simulink model "main_model"  (R2023a)
settings: Solver=ode15s  StartTime=0.0  StopTime=4  FixedStep=0.0001  RelTol=1e-3  AbsTol=1e-3  EnableMultiTasking=on
model workspace (MAT data in the model file):
  C_Gimbal = 0.5
  C_IAP = 0.01
  K_Gimbal = 0
  K_IAP = 200
  a = 1
  b = 1
  muscle_color = [0 0 1]
  muscle_radius = 1
undefined symbols (not defined in the file): X, Y, Z
libraries: nesl_utility x346, sm_lib x329, simulink_extras x33
(part 8 of 11)

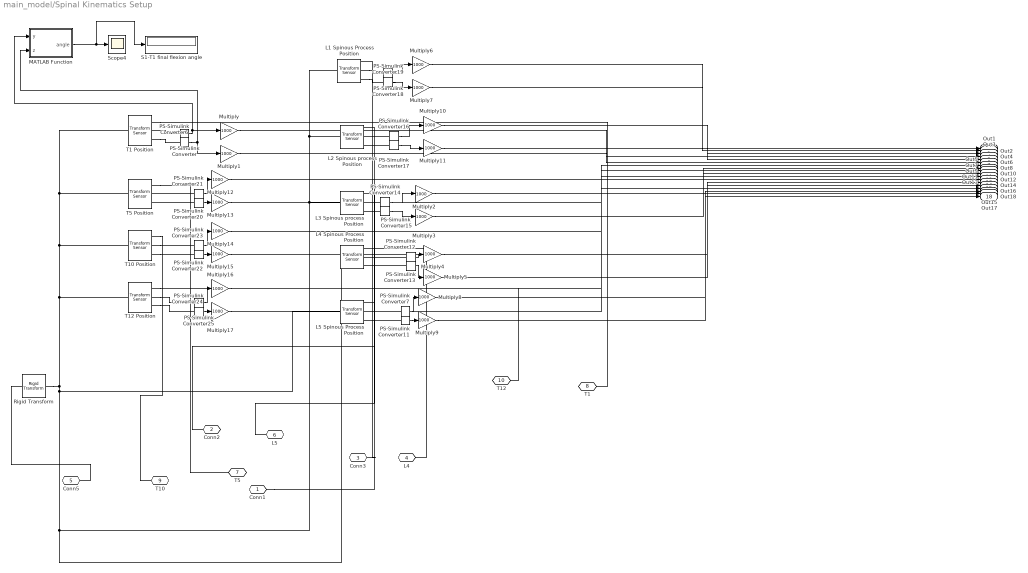
== system main_model/Spinal Kinematics Setup ==
  L1 Spinous Process Position : sm_lib/Frames and Transforms/Transform Sensor  MeasurementFrame=World  RotationSequence=XYX  SenseAngle=off  SenseAxis=off  SenseQ=off  SenseR=off  SenseRotationSequence=off  SenseOmegaX=off  SenseOmegaY=off  SenseOmegaZ=off  SenseQDot=off  SenseRDot=off  SenseRotationSequenceDot=off  SenseAlphaX=off  SenseAlphaY=off  SenseAlphaZ=off  SenseQDDot=off  SenseRDDot=off  SenseX=off  SenseY=on  SenseZ=on  SenseRad=off  SenseAzim=off  SenseDist=off  SenseInc=off  SenseXDot=off  SenseYDot=off  SenseZDot=off  SenseRadDot=off  SenseAzimDot=off  SenseDistDot=off  SenseIncDot=off  SenseXDDot=off  SenseYDDot=off  SenseZDDot=off  SenseRadDDot=off  SenseAzimDDot=off  SenseDistDDot=off  SenseIncDDot=off
  L2 Spinous process Position : sm_lib/Frames and Transforms/Transform Sensor  MeasurementFrame=World  RotationSequence=XYX  SenseAngle=off  SenseAxis=off  SenseQ=off  SenseR=off  SenseRotationSequence=off  SenseOmegaX=off  SenseOmegaY=off  SenseOmegaZ=off  SenseQDot=off  SenseRDot=off  SenseRotationSequenceDot=off  SenseAlphaX=off  SenseAlphaY=off  SenseAlphaZ=off  SenseQDDot=off  SenseRDDot=off  SenseX=off  SenseY=on  SenseZ=on  SenseRad=off  SenseAzim=off  SenseDist=off  SenseInc=off  SenseXDot=off  SenseYDot=off  SenseZDot=off  SenseRadDot=off  SenseAzimDot=off  SenseDistDot=off  SenseIncDot=off  SenseXDDot=off  SenseYDDot=off  SenseZDDot=off  SenseRadDDot=off  SenseAzimDDot=off  SenseDistDDot=off  SenseIncDDot=off
  L3 Spinous process Position : sm_lib/Frames and Transforms/Transform Sensor  MeasurementFrame=World  RotationSequence=XYX  SenseAngle=off  SenseAxis=off  SenseQ=off  SenseR=off  SenseRotationSequence=off  SenseOmegaX=off  SenseOmegaY=off  SenseOmegaZ=off  SenseQDot=off  SenseRDot=off  SenseRotationSequenceDot=off  SenseAlphaX=off  SenseAlphaY=off  SenseAlphaZ=off  SenseQDDot=off  SenseRDDot=off  SenseX=off  SenseY=on  SenseZ=on  SenseRad=off  SenseAzim=off  SenseDist=off  SenseInc=off  SenseXDot=off  SenseYDot=off  SenseZDot=off  SenseRadDot=off  SenseAzimDot=off  SenseDistDot=off  SenseIncDot=off  SenseXDDot=off  SenseYDDot=off  SenseZDDot=off  SenseRadDDot=off  SenseAzimDDot=off  SenseDistDDot=off  SenseIncDDot=off
  L4 Spinous Process Position : sm_lib/Frames and Transforms/Transform Sensor  MeasurementFrame=World  RotationSequence=XYX  SenseAngle=off  SenseAxis=off  SenseQ=off  SenseR=off  SenseRotationSequence=off  SenseOmegaX=off  SenseOmegaY=off  SenseOmegaZ=off  SenseQDot=off  SenseRDot=off  SenseRotationSequenceDot=off  SenseAlphaX=off  SenseAlphaY=off  SenseAlphaZ=off  SenseQDDot=off  SenseRDDot=off  SenseX=off  SenseY=on  SenseZ=on  SenseRad=off  SenseAzim=off  SenseDist=off  SenseInc=off  SenseXDot=off  SenseYDot=off  SenseZDot=off  SenseRadDot=off  SenseAzimDot=off  SenseDistDot=off  SenseIncDot=off  SenseXDDot=off  SenseYDDot=off  SenseZDDot=off  SenseRadDDot=off  SenseAzimDDot=off  SenseDistDDot=off  SenseIncDDot=off
  L5 Spinous Process Position : sm_lib/Frames and Transforms/Transform Sensor  MeasurementFrame=World  RotationSequence=XYX  SenseAngle=off  SenseAxis=off  SenseQ=off  SenseR=off  SenseRotationSequence=off  SenseOmegaX=off  SenseOmegaY=off  SenseOmegaZ=off  SenseQDot=off  SenseRDot=off  SenseRotationSequenceDot=off  SenseAlphaX=off  SenseAlphaY=off  SenseAlphaZ=off  SenseQDDot=off  SenseRDDot=off  SenseX=off  SenseY=on  SenseZ=on  SenseRad=off  SenseAzim=off  SenseDist=off  SenseInc=off  SenseXDot=off  SenseYDot=off  SenseZDot=off  SenseRadDot=off  SenseAzimDot=off  SenseDistDot=off  SenseIncDot=off  SenseXDDot=off  SenseYDDot=off  SenseZDDot=off  SenseRadDDot=off  SenseAzimDDot=off  SenseDistDDot=off  SenseIncDDot=off
  MATLAB Function : MATLAB Function  TreatAsAtomicUnit=on
  Multiply{,1..17} (18 alike) : Gain  Gain=1000
  PS-Simulink Converter{,6..7,11..25} (18 alike) : nesl_utility/PS-Simulink Converter  PhysicalDomain=network_engine_domain  SubClassName=ps_output  LeftPortType=input  RightPortType=output  PseudoPeriodic=off  Frequencies=[]  VectorFormat=inherit  Unit=inherit  AffineConversion=off
  Rigid Transform : sm_lib/Frames and Transforms/Rigid Transform  TranslationMethod=Cartesian  TranslationStandardOffset=0  TranslationStandardOffsetUnits=m  TranslationStandardAxis=+Z  TranslationCartesianOffset=[0 0 0]  TranslationCartesianOffsetUnits=mm  TranslationROffset=0  TranslationROffsetUnits=m  TranslationZOffset=0  TranslationZOffsetUnits=m  TranslationThetaOffset=0  TranslationThetaOffsetUnits=deg  RotationMethod=None  RotationAngleUnits=deg  RotationStandardAxis=+Z  RotationAngle=0.0  RotationArbitraryAxis=[0 0 1]  FollAlignAxisA=+X  BaseAlignAxisA=+Y  FollAlignAxisB=+Y  BaseAlignAxisB=+Z  RotationSequenceAxes=FollowerAxes  RotationSequence=XYX  RotationSequenceAngles=[0 0 0]  RotationSequenceAnglesUnits=deg  RotationMatrix=[1 0 0; 0 1 0; 0 0 1]  Quaternion=[1 0 0 0]
  S1-T1 final flexion angle : Display
  Scope4 : Scope
  T1 Position : sm_lib/Frames and Transforms/Transform Sensor  MeasurementFrame=World  RotationSequence=XYX  SenseAngle=off  SenseAxis=off  SenseQ=off  SenseR=off  SenseRotationSequence=off  SenseOmegaX=off  SenseOmegaY=off  SenseOmegaZ=off  SenseQDot=off  SenseRDot=off  SenseRotationSequenceDot=off  SenseAlphaX=off  SenseAlphaY=off  SenseAlphaZ=off  SenseQDDot=off  SenseRDDot=off  SenseX=off  SenseY=on  SenseZ=on  SenseRad=off  SenseAzim=off  SenseDist=off  SenseInc=off  SenseXDot=off  SenseYDot=off  SenseZDot=off  SenseRadDot=off  SenseAzimDot=off  SenseDistDot=off  SenseIncDot=off  SenseXDDot=off  SenseYDDot=off  SenseZDDot=off  SenseRadDDot=off  SenseAzimDDot=off  SenseDistDDot=off  SenseIncDDot=off
  T10 Position : sm_lib/Frames and Transforms/Transform Sensor  MeasurementFrame=World  RotationSequence=XYX  SenseAngle=off  SenseAxis=off  SenseQ=off  SenseR=off  SenseRotationSequence=off  SenseOmegaX=off  SenseOmegaY=off  SenseOmegaZ=off  SenseQDot=off  SenseRDot=off  SenseRotationSequenceDot=off  SenseAlphaX=off  SenseAlphaY=off  SenseAlphaZ=off  SenseQDDot=off  SenseRDDot=off  SenseX=off  SenseY=on  SenseZ=on  SenseRad=off  SenseAzim=off  SenseDist=off  SenseInc=off  SenseXDot=off  SenseYDot=off  SenseZDot=off  SenseRadDot=off  SenseAzimDot=off  SenseDistDot=off  SenseIncDot=off  SenseXDDot=off  SenseYDDot=off  SenseZDDot=off  SenseRadDDot=off  SenseAzimDDot=off  SenseDistDDot=off  SenseIncDDot=off
  T12 Position : sm_lib/Frames and Transforms/Transform Sensor  MeasurementFrame=World  RotationSequence=XYX  SenseAngle=off  SenseAxis=off  SenseQ=off  SenseR=off  SenseRotationSequence=off  SenseOmegaX=off  SenseOmegaY=off  SenseOmegaZ=off  SenseQDot=off  SenseRDot=off  SenseRotationSequenceDot=off  SenseAlphaX=off  SenseAlphaY=off  SenseAlphaZ=off  SenseQDDot=off  SenseRDDot=off  SenseX=off  SenseY=on  SenseZ=on  SenseRad=off  SenseAzim=off  SenseDist=off  SenseInc=off  SenseXDot=off  SenseYDot=off  SenseZDot=off  SenseRadDot=off  SenseAzimDot=off  SenseDistDot=off  SenseIncDot=off  SenseXDDot=off  SenseYDDot=off  SenseZDDot=off  SenseRadDDot=off  SenseAzimDDot=off  SenseDistDDot=off  SenseIncDDot=off
  T5 Position : sm_lib/Frames and Transforms/Transform Sensor  MeasurementFrame=World  RotationSequence=XYX  SenseAngle=off  SenseAxis=off  SenseQ=off  SenseR=off  SenseRotationSequence=off  SenseOmegaX=off  SenseOmegaY=off  SenseOmegaZ=off  SenseQDot=off  SenseRDot=off  SenseRotationSequenceDot=off  SenseAlphaX=off  SenseAlphaY=off  SenseAlphaZ=off  SenseQDDot=off  SenseRDDot=off  SenseX=off  SenseY=on  SenseZ=on  SenseRad=off  SenseAzim=off  SenseDist=off  SenseInc=off  SenseXDot=off  SenseYDot=off  SenseZDot=off  SenseRadDot=off  SenseAzimDot=off  SenseDistDot=off  SenseIncDot=off  SenseXDDot=off  SenseYDDot=off  SenseZDDot=off  SenseRadDDot=off  SenseAzimDDot=off  SenseDistDDot=off  SenseIncDDot=off
  Conn1 : PMIOPort  Side=Right
  Conn2 : PMIOPort  Port=2  Side=Right
  Conn3 : PMIOPort  Port=3  Side=Right
  L4 : PMIOPort  Port=4  Side=Right
  Conn5 : PMIOPort  Port=5  Side=Left
  L5 : PMIOPort  Port=6  Side=Right
  T5 : PMIOPort  Port=7  Side=Right
  T1 : PMIOPort  Port=8  Side=Right
  T10 : PMIOPort  Port=9  Side=Right
  T12 : PMIOPort  Port=10  Side=Right
  Out1 : Outport
  Out2 : Outport  Port=2
  Out3 : Outport  Port=3
  Out4 : Outport  Port=4
  Out5 : Outport  Port=5
  Out6 : Outport  Port=6
  Out7 : Outport  Port=7
  Out8 : Outport  Port=8
  Out9 : Outport  Port=9
  Out10 : Outport  Port=10
  Out11 : Outport  Port=11
  Out12 : Outport  Port=12
  Out13 : Outport  Port=13
  Out14 : Outport  Port=14
  Out15 : Outport  Port=15
  Out16 : Outport  Port=16
  Out17 : Outport  Port=17
  Out18 : Outport  Port=18
  wires:
  Multiply9/1 -> Out18/1
  Multiply17/1 -> Out17/1
  Multiply5/1 -> Out14/1
  Multiply12/1 -> Out7/1
  Multiply2/1 -> Out8/1
  Multiply10/1 -> Out3/1
  Multiply13/1 -> Out9/1
  Multiply6/1 -> Out1/1
  Multiply4/1 -> Out13/1
  PS-Simulink Converter7/1 -> Multiply8/1
  PS-Simulink Converter13/1 -> Multiply5/1
  Multiply11/1 -> Out5/1
  Multiply8/1 -> Out16/1
  Multiply/1 -> Out4/1
  Multiply16/1 -> Out15/1
  PS-Simulink Converter24/1 -> Multiply17/1
  Multiply15/1 -> Out12/1
  Multiply7/1 -> Out2/1
  PS-Simulink Converter22/1 -> Multiply15/1
  PS-Simulink Converter23/1 -> Multiply14/1
  PS-Simulink Converter15/1 -> Multiply3/1
  PS-Simulink Converter20/1 -> Multiply13/1
  PS-Simulink Converter11/1 -> Multiply9/1
  PS-Simulink Converter14/1 -> Multiply2/1
  Multiply14/1 -> Out11/1
  PS-Simulink Converter21/1 -> Multiply12/1
  PS-Simulink Converter18/1 -> Multiply6/1
  Multiply1/1 -> Out6/1
  PS-Simulink Converter16/1 -> Multiply10/1
  PS-Simulink Converter17/1 -> Multiply11/1
  Multiply3/1 -> Out10/1
  PS-Simulink Converter25/1 -> Multiply16/1
  PS-Simulink Converter12/1 -> Multiply4/1
  PS-Simulink Converter19/1 -> Multiply7/1
  MATLAB Function/1(angle) -> Scope4/1, S1-T1 final flexion angle/1
  PS-Simulink Converter/1 -> MATLAB Function/1(y), Multiply/1
  PS-Simulink Converter6/1 -> Multiply1/1, MATLAB Function/2(z)
  connections:
  L4 Spinous Process Position/RConn1 -- L4/RConn1
  T10 Position/RConn1 -- T10/RConn1
  L1 Spinous Process Position/RConn2 -- PS-Simulink Converter18/LConn1
  T5 Position/RConn1 -- T5/RConn1
  PS-Simulink Converter21/LConn1 -- T5 Position/RConn2
  L3 Spinous process Position/RConn2 -- PS-Simulink Converter14/LConn1
  T10 Position/RConn3 -- PS-Simulink Converter22/LConn1
  T1 Position/RConn3 -- PS-Simulink Converter6/LConn1
  PS-Simulink Converter20/LConn1 -- T5 Position/RConn3
  Conn1/RConn1 -- L2 Spinous process Position/RConn1
  L1 Spinous Process Position/RConn3 -- PS-Simulink Converter19/LConn1
  Rigid Transform/LConn1 -- Conn5/RConn1
  L2 Spinous process Position/RConn3 -- PS-Simulink Converter17/LConn1
  T1 Position/RConn2 -- PS-Simulink Converter/LConn1
  L5 Spinous Process Position/RConn1 -- L5/RConn1
  T10 Position/RConn2 -- PS-Simulink Converter23/LConn1
  L5 Spinous Process Position/RConn2 -- PS-Simulink Converter7/LConn1
  L3 Spinous process Position/RConn1 -- Conn2/RConn1
  T12 Position/RConn3 -- PS-Simulink Converter24/LConn1
  T12 Position/RConn2 -- PS-Simulink Converter25/LConn1
  Conn3/RConn1 -- L1 Spinous Process Position/RConn1
  L4 Spinous Process Position/LConn1 -- L3 Spinous process Position/LConn1 -- L2 Spinous process Position/LConn1 -- L1 Spinous Process Position/LConn1 -- L5 Spinous Process Position/LConn1 -- Rigid Transform/RConn1 -- T12 Position/LConn1 -- T10 Position/LConn1 -- T5 Position/LConn1 -- T1 Position/LConn1
  L5 Spinous Process Position/RConn3 -- PS-Simulink Converter11/LConn1
  L3 Spinous process Position/RConn3 -- PS-Simulink Converter15/LConn1
  T1 Position/RConn1 -- T1/RConn1
  L4 Spinous Process Position/RConn2 -- PS-Simulink Converter12/LConn1
  T12 Position/RConn1 -- T12/RConn1
  L4 Spinous Process Position/RConn3 -- PS-Simulink Converter13/LConn1
  L2 Spinous process Position/RConn2 -- PS-Simulink Converter16/LConn1

== system main_model/L1/AR torque feedback L4 ==
  Constant : Constant  Value=0.7
  Constant1 : Constant  Value=0.7
  Gain5 : Gain  Gain=-1
  PS-Simulink Converter9 : nesl_utility/PS-Simulink Converter  PhysicalDomain=network_engine_domain  SubClassName=ps_output  LeftPortType=input  RightPortType=output  PseudoPeriodic=off  Frequencies=[]  VectorFormat=1-D array  Unit=inherit  AffineConversion=off
  Radians to Degrees : simulink_extras/Transformations/Radians to Degrees
  Simulink-PS Converter6 : nesl_utility/Simulink-PS Converter  PhysicalDomain=network_engine_domain  SubClassName=ps_input  LeftPortType=input  RightPortType=output  PseudoPeriodic=off  Frequencies=[]  NoiseDistribution=none  NoiseParameters=[]  Unit=1  AffineConversion=off  FilteringAndDerivatives=provide  SimscapeFilterOrder=1  InputFilterTimeConstant=0.001  UdotUserProvided=0
  peacewise torque profile5 : MATLAB Function  TreatAsAtomicUnit=on
  AR rot : PMIOPort  Side=Left
  AR torque : PMIOPort  Port=2  Side=Right
  wires:
  Constant1/1 -> peacewise torque profile5/3(b)
  Constant/1 -> peacewise torque profile5/2(a)
  Radians to Degrees/1 -> peacewise torque profile5/1(u)
  Gain5/1 -> Simulink-PS Converter6/1
  peacewise torque profile5/1(torque) -> Gain5/1
  PS-Simulink Converter9/1 -> Radians to Degrees/1
  connections:
  AR torque/RConn1 -- Simulink-PS Converter6/RConn1
  PS-Simulink Converter9/LConn1 -- AR rot/RConn1

== system main_model/L1/FE torque feedback L4 ==
  Constant : Constant  Value=a
  Constant1 : Constant  Value=b
  Gain1 : Gain  Gain=-1
  Gain7 : Gain
  PS-Simulink Converter5 : nesl_utility/PS-Simulink Converter  PhysicalDomain=network_engine_domain  SubClassName=ps_output  LeftPortType=input  RightPortType=output  PseudoPeriodic=off  Frequencies=[]  VectorFormat=1-D array  Unit=inherit  AffineConversion=off
  Radians to Degrees : simulink_extras/Transformations/Radians to Degrees
  Simulink-PS Converter4 : nesl_utility/Simulink-PS Converter  PhysicalDomain=network_engine_domain  SubClassName=ps_input  LeftPortType=input  RightPortType=output  PseudoPeriodic=off  Frequencies=[]  NoiseDistribution=none  NoiseParameters=[]  Unit=1  AffineConversion=off  FilteringAndDerivatives=provide  SimscapeFilterOrder=1  InputFilterTimeConstant=0.001  UdotUserProvided=0
  peacewise torque profile1 : MATLAB Function  TreatAsAtomicUnit=on
  FE rot : PMIOPort  Side=Left
  FE torque : PMIOPort  Port=2  Side=Right
  wires:
  Constant1/1 -> peacewise torque profile1/3(b)
  Constant/1 -> peacewise torque profile1/2(a)
  Gain1/1 -> peacewise torque profile1/1(u)
  Radians to Degrees/1 -> Gain1/1
  Gain7/1 -> Simulink-PS Converter4/1
  peacewise torque profile1/1(torque) -> Gain7/1
  PS-Simulink Converter5/1 -> Radians to Degrees/1
  connections:
  FE torque/RConn1 -- Simulink-PS Converter4/RConn1
  FE rot/RConn1 -- PS-Simulink Converter5/LConn1

== system main_model/L1/LB torque feedback L4 ==
  Constant : Constant  Value=a
  Constant1 : Constant  Value=b
  Gain4 : Gain  Gain=-1
  PS-Simulink Converter8 : nesl_utility/PS-Simulink Converter  PhysicalDomain=network_engine_domain  SubClassName=ps_output  LeftPortType=input  RightPortType=output  PseudoPeriodic=off  Frequencies=[]  VectorFormat=1-D array  Unit=inherit  AffineConversion=off
  Radians to Degrees : simulink_extras/Transformations/Radians to Degrees
  Simulink-PS Converter5 : nesl_utility/Simulink-PS Converter  PhysicalDomain=network_engine_domain  SubClassName=ps_input  LeftPortType=input  RightPortType=output  PseudoPeriodic=off  Frequencies=[]  NoiseDistribution=none  NoiseParameters=[]  Unit=1  AffineConversion=off  FilteringAndDerivatives=provide  SimscapeFilterOrder=1  InputFilterTimeConstant=0.001  UdotUserProvided=0
  peacewise torque profile4 : MATLAB Function  TreatAsAtomicUnit=on
  LB rot : PMIOPort  Side=Left
  LB torque : PMIOPort  Port=2  Side=Right
  wires:
  Radians to Degrees/1 -> peacewise torque profile4/1(u)
  Constant1/1 -> peacewise torque profile4/3(b)
  Constant/1 -> peacewise torque profile4/2(a)
  peacewise torque profile4/1(torque) -> Gain4/1
  PS-Simulink Converter8/1 -> Radians to Degrees/1
  Gain4/1 -> Simulink-PS Converter5/1
  connections:
  LB rot/RConn1 -- PS-Simulink Converter8/LConn1
  Simulink-PS Converter5/RConn1 -- LB torque/RConn1

== system main_model/L2/AR torque feedback L4 ==
  Constant : Constant  Value=0.7
  Constant1 : Constant  Value=0.7
  Gain5 : Gain  Gain=-1
  PS-Simulink Converter9 : nesl_utility/PS-Simulink Converter  PhysicalDomain=network_engine_domain  SubClassName=ps_output  LeftPortType=input  RightPortType=output  PseudoPeriodic=off  Frequencies=[]  VectorFormat=1-D array  Unit=inherit  AffineConversion=off
  Radians to Degrees : simulink_extras/Transformations/Radians to Degrees
  Simulink-PS Converter6 : nesl_utility/Simulink-PS Converter  PhysicalDomain=network_engine_domain  SubClassName=ps_input  LeftPortType=input  RightPortType=output  PseudoPeriodic=off  Frequencies=[]  NoiseDistribution=none  NoiseParameters=[]  Unit=1  AffineConversion=off  FilteringAndDerivatives=provide  SimscapeFilterOrder=1  InputFilterTimeConstant=0.001  UdotUserProvided=0
  peacewise torque profile5 : MATLAB Function  TreatAsAtomicUnit=on
  AR rot : PMIOPort  Side=Left
  AR torque : PMIOPort  Port=2  Side=Right
  wires:
  Constant1/1 -> peacewise torque profile5/3(b)
  Constant/1 -> peacewise torque profile5/2(a)
  Radians to Degrees/1 -> peacewise torque profile5/1(u)
  PS-Simulink Converter9/1 -> Radians to Degrees/1
  peacewise torque profile5/1(torque) -> Gain5/1
  Gain5/1 -> Simulink-PS Converter6/1
  connections:
  PS-Simulink Converter9/LConn1 -- AR rot/RConn1
  AR torque/RConn1 -- Simulink-PS Converter6/RConn1

== system main_model/L2/FE torque feedback L4 ==
  Constant : Constant  Value=a
  Constant1 : Constant  Value=b
  Gain1 : Gain  Gain=-1
  Gain7 : Gain
  PS-Simulink Converter5 : nesl_utility/PS-Simulink Converter  PhysicalDomain=network_engine_domain  SubClassName=ps_output  LeftPortType=input  RightPortType=output  PseudoPeriodic=off  Frequencies=[]  VectorFormat=1-D array  Unit=inherit  AffineConversion=off
  Radians to Degrees : simulink_extras/Transformations/Radians to Degrees
  Simulink-PS Converter4 : nesl_utility/Simulink-PS Converter  PhysicalDomain=network_engine_domain  SubClassName=ps_input  LeftPortType=input  RightPortType=output  PseudoPeriodic=off  Frequencies=[]  NoiseDistribution=none  NoiseParameters=[]  Unit=1  AffineConversion=off  FilteringAndDerivatives=provide  SimscapeFilterOrder=1  InputFilterTimeConstant=0.001  UdotUserProvided=0
  peacewise torque profile1 : MATLAB Function  TreatAsAtomicUnit=on
  FE rot : PMIOPort  Side=Left
  FE torque : PMIOPort  Port=2  Side=Right
  wires:
  Gain1/1 -> peacewise torque profile1/1(u)
  Constant1/1 -> peacewise torque profile1/3(b)
  Constant/1 -> peacewise torque profile1/2(a)
  PS-Simulink Converter5/1 -> Radians to Degrees/1
  Radians to Degrees/1 -> Gain1/1
  peacewise torque profile1/1(torque) -> Gain7/1
  Gain7/1 -> Simulink-PS Converter4/1
  connections:
  FE rot/RConn1 -- PS-Simulink Converter5/LConn1
  FE torque/RConn1 -- Simulink-PS Converter4/RConn1

== system main_model/L2/LB torque feedback L4 ==
  Constant : Constant  Value=a
  Constant1 : Constant  Value=b
  Gain4 : Gain  Gain=-1
  PS-Simulink Converter8 : nesl_utility/PS-Simulink Converter  PhysicalDomain=network_engine_domain  SubClassName=ps_output  LeftPortType=input  RightPortType=output  PseudoPeriodic=off  Frequencies=[]  VectorFormat=1-D array  Unit=inherit  AffineConversion=off
  Radians to Degrees : simulink_extras/Transformations/Radians to Degrees
  Simulink-PS Converter5 : nesl_utility/Simulink-PS Converter  PhysicalDomain=network_engine_domain  SubClassName=ps_input  LeftPortType=input  RightPortType=output  PseudoPeriodic=off  Frequencies=[]  NoiseDistribution=none  NoiseParameters=[]  Unit=1  AffineConversion=off  FilteringAndDerivatives=provide  SimscapeFilterOrder=1  InputFilterTimeConstant=0.001  UdotUserProvided=0
  peacewise torque profile4 : MATLAB Function  TreatAsAtomicUnit=on
  LB rot : PMIOPort  Side=Left
  LB torque : PMIOPort  Port=2  Side=Right
  wires:
  Radians to Degrees/1 -> peacewise torque profile4/1(u)
  Constant1/1 -> peacewise torque profile4/3(b)
  Constant/1 -> peacewise torque profile4/2(a)
  Gain4/1 -> Simulink-PS Converter5/1
  PS-Simulink Converter8/1 -> Radians to Degrees/1
  peacewise torque profile4/1(torque) -> Gain4/1
  connections:
  Simulink-PS Converter5/RConn1 -- LB torque/RConn1
  LB rot/RConn1 -- PS-Simulink Converter8/LConn1

== system main_model/L3/AR torque feedback L4 ==
  Constant : Constant  Value=0.7
  Constant1 : Constant  Value=0.7
  Gain5 : Gain  Gain=-1
  PS-Simulink Converter9 : nesl_utility/PS-Simulink Converter  PhysicalDomain=network_engine_domain  SubClassName=ps_output  LeftPortType=input  RightPortType=output  PseudoPeriodic=off  Frequencies=[]  VectorFormat=1-D array  Unit=inherit  AffineConversion=off
  Radians to Degrees : simulink_extras/Transformations/Radians to Degrees
  Simulink-PS Converter6 : nesl_utility/Simulink-PS Converter  PhysicalDomain=network_engine_domain  SubClassName=ps_input  LeftPortType=input  RightPortType=output  PseudoPeriodic=off  Frequencies=[]  NoiseDistribution=none  NoiseParameters=[]  Unit=1  AffineConversion=off  FilteringAndDerivatives=provide  SimscapeFilterOrder=1  InputFilterTimeConstant=0.001  UdotUserProvided=0
  peacewise torque profile5 : MATLAB Function  TreatAsAtomicUnit=on
  AR rot : PMIOPort  Side=Left
  AR torque : PMIOPort  Port=2  Side=Right
  wires:
  Constant1/1 -> peacewise torque profile5/3(b)
  Constant/1 -> peacewise torque profile5/2(a)
  Radians to Degrees/1 -> peacewise torque profile5/1(u)
  PS-Simulink Converter9/1 -> Radians to Degrees/1
  Gain5/1 -> Simulink-PS Converter6/1
  peacewise torque profile5/1(torque) -> Gain5/1
  connections:
  AR torque/RConn1 -- Simulink-PS Converter6/RConn1
  PS-Simulink Converter9/LConn1 -- AR rot/RConn1

== system main_model/L3/FE torque feedback L4 ==
  Constant : Constant  Value=a
  Constant1 : Constant  Value=b
  Gain1 : Gain  Gain=-1
  Gain7 : Gain
  PS-Simulink Converter5 : nesl_utility/PS-Simulink Converter  PhysicalDomain=network_engine_domain  SubClassName=ps_output  LeftPortType=input  RightPortType=output  PseudoPeriodic=off  Frequencies=[]  VectorFormat=1-D array  Unit=inherit  AffineConversion=off
  Radians to Degrees : simulink_extras/Transformations/Radians to Degrees
  Simulink-PS Converter4 : nesl_utility/Simulink-PS Converter  PhysicalDomain=network_engine_domain  SubClassName=ps_input  LeftPortType=input  RightPortType=output  PseudoPeriodic=off  Frequencies=[]  NoiseDistribution=none  NoiseParameters=[]  Unit=1  AffineConversion=off  FilteringAndDerivatives=provide  SimscapeFilterOrder=1  InputFilterTimeConstant=0.001  UdotUserProvided=0
  peacewise torque profile1 : MATLAB Function  TreatAsAtomicUnit=on
  FE rot : PMIOPort  Side=Left
  FE torque : PMIOPort  Port=2  Side=Right
  wires:
  Gain1/1 -> peacewise torque profile1/1(u)
  Constant1/1 -> peacewise torque profile1/3(b)
  Constant/1 -> peacewise torque profile1/2(a)
  PS-Simulink Converter5/1 -> Radians to Degrees/1
  Radians to Degrees/1 -> Gain1/1
  Gain7/1 -> Simulink-PS Converter4/1
  peacewise torque profile1/1(torque) -> Gain7/1
  connections:
  FE torque/RConn1 -- Simulink-PS Converter4/RConn1
  FE rot/RConn1 -- PS-Simulink Converter5/LConn1

== system main_model/L3/LB torque feedback L4 ==
  Constant : Constant  Value=a
  Constant1 : Constant  Value=b
  Gain4 : Gain  Gain=-1
  PS-Simulink Converter8 : nesl_utility/PS-Simulink Converter  PhysicalDomain=network_engine_domain  SubClassName=ps_output  LeftPortType=input  RightPortType=output  PseudoPeriodic=off  Frequencies=[]  VectorFormat=1-D array  Unit=inherit  AffineConversion=off
  Radians to Degrees : simulink_extras/Transformations/Radians to Degrees
  Simulink-PS Converter5 : nesl_utility/Simulink-PS Converter  PhysicalDomain=network_engine_domain  SubClassName=ps_input  LeftPortType=input  RightPortType=output  PseudoPeriodic=off  Frequencies=[]  NoiseDistribution=none  NoiseParameters=[]  Unit=1  AffineConversion=off  FilteringAndDerivatives=provide  SimscapeFilterOrder=1  InputFilterTimeConstant=0.001  UdotUserProvided=0
  peacewise torque profile4 : MATLAB Function  TreatAsAtomicUnit=on
  LB rot : PMIOPort  Side=Left
  LB torque : PMIOPort  Port=2  Side=Right
  wires:
  Radians to Degrees/1 -> peacewise torque profile4/1(u)
  Constant1/1 -> peacewise torque profile4/3(b)
  Constant/1 -> peacewise torque profile4/2(a)
  peacewise torque profile4/1(torque) -> Gain4/1
  PS-Simulink Converter8/1 -> Radians to Degrees/1
  Gain4/1 -> Simulink-PS Converter5/1
  connections:
  LB rot/RConn1 -- PS-Simulink Converter8/LConn1
  Simulink-PS Converter5/RConn1 -- LB torque/RConn1

== system main_model/L4/AR torque feedback L4 ==
  Constant : Constant  Value=0.7
  Constant1 : Constant  Value=0.7
  Gain5 : Gain  Gain=-1
  PS-Simulink Converter9 : nesl_utility/PS-Simulink Converter  PhysicalDomain=network_engine_domain  SubClassName=ps_output  LeftPortType=input  RightPortType=output  PseudoPeriodic=off  Frequencies=[]  VectorFormat=1-D array  Unit=inherit  AffineConversion=off
  Radians to Degrees : simulink_extras/Transformations/Radians to Degrees
  Simulink-PS Converter6 : nesl_utility/Simulink-PS Converter  PhysicalDomain=network_engine_domain  SubClassName=ps_input  LeftPortType=input  RightPortType=output  PseudoPeriodic=off  Frequencies=[]  NoiseDistribution=none  NoiseParameters=[]  Unit=1  AffineConversion=off  FilteringAndDerivatives=provide  SimscapeFilterOrder=1  InputFilterTimeConstant=0.001  UdotUserProvided=0
  peacewise torque profile5 : MATLAB Function  TreatAsAtomicUnit=on
  AR rot : PMIOPort  Side=Left
  AR torque : PMIOPort  Port=2  Side=Right
  wires:
  Constant1/1 -> peacewise torque profile5/3(b)
  Constant/1 -> peacewise torque profile5/2(a)
  Radians to Degrees/1 -> peacewise torque profile5/1(u)
  PS-Simulink Converter9/1 -> Radians to Degrees/1
  peacewise torque profile5/1(torque) -> Gain5/1
  Gain5/1 -> Simulink-PS Converter6/1
  connections:
  PS-Simulink Converter9/LConn1 -- AR rot/RConn1
  AR torque/RConn1 -- Simulink-PS Converter6/RConn1

== system main_model/L4/FE torque feedback L4 ==
  Constant : Constant  Value=a
  Constant1 : Constant  Value=b
  Gain1 : Gain  Gain=-1
  Gain7 : Gain
  PS-Simulink Converter5 : nesl_utility/PS-Simulink Converter  PhysicalDomain=network_engine_domain  SubClassName=ps_output  LeftPortType=input  RightPortType=output  PseudoPeriodic=off  Frequencies=[]  VectorFormat=1-D array  Unit=inherit  AffineConversion=off
  Radians to Degrees : simulink_extras/Transformations/Radians to Degrees
  Scope : Scope  NumInputPorts=2
  Simulink-PS Converter4 : nesl_utility/Simulink-PS Converter  PhysicalDomain=network_engine_domain  SubClassName=ps_input  LeftPortType=input  RightPortType=output  PseudoPeriodic=off  Frequencies=[]  NoiseDistribution=none  NoiseParameters=[]  Unit=1  AffineConversion=off  FilteringAndDerivatives=provide  SimscapeFilterOrder=1  InputFilterTimeConstant=0.001  UdotUserProvided=0
  peacewise torque profile1 : MATLAB Function  TreatAsAtomicUnit=on
  FE rot : PMIOPort  Side=Left
  FE torque : PMIOPort  Port=2  Side=Right
  wires:
  Gain1/1 -> peacewise torque profile1/1(u), Scope/1
  Constant1/1 -> peacewise torque profile1/3(b)
  Constant/1 -> peacewise torque profile1/2(a)
  PS-Simulink Converter5/1 -> Radians to Degrees/1
  Radians to Degrees/1 -> Gain1/1
  peacewise torque profile1/1(torque) -> Gain7/1
  Gain7/1 -> Simulink-PS Converter4/1, Scope/2
  connections:
  FE rot/RConn1 -- PS-Simulink Converter5/LConn1
  FE torque/RConn1 -- Simulink-PS Converter4/RConn1

== system main_model/L4/LB torque feedback L4 ==
  Constant : Constant  Value=a
  Constant1 : Constant  Value=b
  Gain4 : Gain  Gain=-1
  PS-Simulink Converter8 : nesl_utility/PS-Simulink Converter  PhysicalDomain=network_engine_domain  SubClassName=ps_output  LeftPortType=input  RightPortType=output  PseudoPeriodic=off  Frequencies=[]  VectorFormat=1-D array  Unit=inherit  AffineConversion=off
  Radians to Degrees : simulink_extras/Transformations/Radians to Degrees
  Simulink-PS Converter5 : nesl_utility/Simulink-PS Converter  PhysicalDomain=network_engine_domain  SubClassName=ps_input  LeftPortType=input  RightPortType=output  PseudoPeriodic=off  Frequencies=[]  NoiseDistribution=none  NoiseParameters=[]  Unit=1  AffineConversion=off  FilteringAndDerivatives=provide  SimscapeFilterOrder=1  InputFilterTimeConstant=0.001  UdotUserProvided=0
  peacewise torque profile4 : MATLAB Function  TreatAsAtomicUnit=on
  LB rot : PMIOPort  Side=Left
  LB torque : PMIOPort  Port=2  Side=Right
  wires:
  Radians to Degrees/1 -> peacewise torque profile4/1(u)
  Constant1/1 -> peacewise torque profile4/3(b)
  Constant/1 -> peacewise torque profile4/2(a)
  Gain4/1 -> Simulink-PS Converter5/1
  PS-Simulink Converter8/1 -> Radians to Degrees/1
  peacewise torque profile4/1(torque) -> Gain4/1
  connections:
  Simulink-PS Converter5/RConn1 -- LB torque/RConn1
  LB rot/RConn1 -- PS-Simulink Converter8/LConn1

== system main_model/L5/AR torque feedback L5 ==
  Constant : Constant  Value=0.7
  Constant1 : Constant  Value=0.7
  Gain2 : Gain  Gain=-1
  PS-Simulink Converter3 : nesl_utility/PS-Simulink Converter  PhysicalDomain=network_engine_domain  SubClassName=ps_output  LeftPortType=input  RightPortType=output  PseudoPeriodic=off  Frequencies=[]  VectorFormat=1-D array  Unit=inherit  AffineConversion=off
  Radians to Degrees : simulink_extras/Transformations/Radians to Degrees
  Simulink-PS Converter2 : nesl_utility/Simulink-PS Converter  PhysicalDomain=network_engine_domain  SubClassName=ps_input  LeftPortType=input  RightPortType=output  PseudoPeriodic=off  Frequencies=[]  NoiseDistribution=none  NoiseParameters=[]  Unit=1  AffineConversion=off  FilteringAndDerivatives=provide  SimscapeFilterOrder=1  InputFilterTimeConstant=0.001  UdotUserProvided=0
  peacewise torque profile3 : MATLAB Function  TreatAsAtomicUnit=on
  AR rot : PMIOPort  Side=Left
  AR torque : PMIOPort  Port=2  Side=Right
  wires:
  Constant1/1 -> peacewise torque profile3/3(b)
  Constant/1 -> peacewise torque profile3/2(a)
  Radians to Degrees/1 -> peacewise torque profile3/1(u)
  PS-Simulink Converter3/1 -> Radians to Degrees/1
  Gain2/1 -> Simulink-PS Converter2/1
  peacewise torque profile3/1(torque) -> Gain2/1
  connections:
  PS-Simulink Converter3/LConn1 -- AR rot/RConn1
  AR torque/RConn1 -- Simulink-PS Converter2/RConn1

== system main_model/L5/FE torque feedback L5 ==
  Constant : Constant  Value=a
  Constant1 : Constant  Value=b
  Gain1 : Gain  Gain=-1
  Gain6 : Gain
  PS-Simulink Converter : nesl_utility/PS-Simulink Converter  PhysicalDomain=network_engine_domain  SubClassName=ps_output  LeftPortType=input  RightPortType=output  PseudoPeriodic=off  Frequencies=[]  VectorFormat=inherit  Unit=inherit  AffineConversion=off
  Radians to Degrees : simulink_extras/Transformations/Radians to Degrees
  Scope : Scope  NumInputPorts=2
  Simulink-PS Converter3 : nesl_utility/Simulink-PS Converter  PhysicalDomain=network_engine_domain  SubClassName=ps_input  LeftPortType=input  RightPortType=output  PseudoPeriodic=off  Frequencies=[]  NoiseDistribution=none  NoiseParameters=[]  Unit=1  AffineConversion=off  FilteringAndDerivatives=provide  SimscapeFilterOrder=1  InputFilterTimeConstant=0.001  UdotUserProvided=0
  XY Graph : Record  FileSettingsInternal="{\"entries\":[{\"content\":{\"excelSettings\":{\"content\":{},\"type\":\"Streamout.ExcelSettings\"}},\"type\":\"Streamout.FileSettingStorage\",\"uuid\":\"21849821-9f95-4fe4-8d79-13356bbc0b36\"}],\"packageUris\":[\"http://schema.mathworks.com/mf0/streamout_blocks/R2020a\"],\"version\":\"1.0\"}"  Layout=[1 1]  SignalsInternal="{\"entries\":[{\"content\":{\"signals\":[{\"content\":{\"blockPath\":[\"main_model/L5/FE torque feedback L5/XY Graph\"],\"dimensions\":[1],\"domain\":\"main_model/L5/FE torque feedback L5/XY Graph\",\"lineColor\":\"#4dbeee\",\"port\":1,\"signalID\":1772,\"signalName\":\"moment\"},\"type\":\"RecordBlkView.Signal\",\"uuid\":\"63c73282-42d9-4aea-a135-8bf1856202d8\"},{\"content\":{\"blockPath\":[\"main_model/L5/FE torque feedback L5/XY Graph\"],\"dimensions\":[1,1],\"domain\":\"main_model/L5/FE torque feedback L5/XY Graph\",\"lineColor\":\"#a2142f\",\"port\":2,\"signalID\":1775,\"signalName\":\"rot\"},\"type\":\"RecordBlkView.Signal\",\"uuid\":\"2cce2bc2-92f3-4c7e-868c-ac92c3e97ccb\"}]},\"type\":\"RecordBlkView.InputSignals\",\"uuid\":\"b0d75595-b0eb-49bf-926c-fd4db05ca047\"}],\"packageUris\":[\"http://schema.mathworks.com/mf0/streamout_blocks/R2020a\"],\"version\":\"1.0\"}"  VisualizationBindings="{\"xyplotplugin\":{\"info\":[{\"series\":[],\"subplotID\":1}]}}"  CompatibilityTag=XY
  peacewise torque profile (+- 15 deg) : MATLAB Function  TreatAsAtomicUnit=on
  FE torque : PMIOPort  Side=Right
  FE rot : PMIOPort  Port=2  Side=Left
  wires:
  Gain1/1 -> peacewise torque profile (+- 15 deg)/1(u), Scope/2, XY Graph/2  "rot"
  Constant1/1 -> peacewise torque profile (+- 15 deg)/3(b)
  Constant/1 -> peacewise torque profile (+- 15 deg)/2(a)
  PS-Simulink Converter/1 -> Radians to Degrees/1
  Radians to Degrees/1 -> Gain1/1
  peacewise torque profile (+- 15 deg)/1(torque) -> Gain6/1
  Gain6/1 -> Simulink-PS Converter3/1, Scope/1, XY Graph/1  "moment"
  connections:
  Simulink-PS Converter3/RConn1 -- FE torque/RConn1
  FE rot/RConn1 -- PS-Simulink Converter/LConn1

== system main_model/L5/LB torque feedback L5 ==
  Constant : Constant  Value=a
  Constant1 : Constant  Value=b
  Gain1 : Gain  Gain=-1
  PS-Simulink Converter2 : nesl_utility/PS-Simulink Converter  PhysicalDomain=network_engine_domain  SubClassName=ps_output  LeftPortType=input  RightPortType=output  PseudoPeriodic=off  Frequencies=[]  VectorFormat=1-D array  Unit=inherit  AffineConversion=off
  Radians to Degrees : simulink_extras/Transformations/Radians to Degrees
  Simulink-PS Converter1 : nesl_utility/Simulink-PS Converter  PhysicalDomain=network_engine_domain  SubClassName=ps_input  LeftPortType=input  RightPortType=output  PseudoPeriodic=off  Frequencies=[]  NoiseDistribution=none  NoiseParameters=[]  Unit=1  AffineConversion=off  FilteringAndDerivatives=provide  SimscapeFilterOrder=1  InputFilterTimeConstant=0.001  UdotUserProvided=0
  peacewise torque profile2 : MATLAB Function  TreatAsAtomicUnit=on
  LB rot : PMIOPort  Side=Left
  LB torque : PMIOPort  Port=2  Side=Right
  wires:
  Radians to Degrees/1 -> peacewise torque profile2/1(u)
  Constant1/1 -> peacewise torque profile2/3(b)
  Constant/1 -> peacewise torque profile2/2(a)
  peacewise torque profile2/1(torque) -> Gain1/1
  PS-Simulink Converter2/1 -> Radians to Degrees/1
  Gain1/1 -> Simulink-PS Converter1/1
  connections:
  Simulink-PS Converter1/RConn1 -- LB torque/RConn1
  LB rot/RConn1 -- PS-Simulink Converter2/LConn1

== system main_model/Muscle Forces setup/Muscle1 ==
  Constant : Constant  Value=0
  Constant1 : Constant  Value=0
  Gimbal Joint : sm_lib/Joints/Gimbal Joint  JointMode=Normal  SenseConstraintForce=off  SenseConstraintForceX=off  SenseConstraintForceY=off  SenseConstraintForceZ=off  SenseConstraintTorque=off  SenseConstraintTorqueX=off  SenseConstraintTorqueY=off  SenseConstraintTorqueZ=off  SenseTotalForce=off  SenseTotalForceX=off  SenseTotalForceY=off  SenseTotalForceZ=off  SenseTotalTorque=off  SenseTotalTorqueX=off  SenseTotalTorqueY=off  SenseTotalTorqueZ=off  CompositeWrenchDir=FollowerOnBase  CompositeWrenchFrame=BaseFrame  RxEquilibriumPosition=0  RxEquilibriumPositionUnits=deg  RxSpringStiffness=0  RxSpringStiffnessUnits=N*m/deg  RxDampingCoefficient=0  RxDampingCoefficientUnits=N*m/(deg/s)  RxTorqueActuationMode=ComputedTorque  RxMotionActuationMode=InputMotion  RxSensePosition=off  RxSenseVelocity=off  RxSenseAcceleration=off  RxSenseTorqueForce=off  RxSenseLowerLimitTorqueForce=off  RxSenseUpperLimitTorqueForce=off  RxLowerLimitSpecify=off  RxLowerLimitBound=-90  RxLowerLimitBoundUnits=deg  RxLowerLimitStiffness=1e4  RxLowerLimitStiffnessUnits=N*m/deg  RxLowerLimitDamping=10  RxLowerLimitDampingUnits=N*m/(deg/s)  RxLowerLimitTransitionRegionWidth=0.1  RxLowerLimitTransitionRegionWidthUnits=deg  RxUpperLimitSpecify=off  RxUpperLimitBound=90  RxUpperLimitBoundUnits=deg  RxUpperLimitStiffness=1e4  RxUpperLimitStiffnessUnits=N*m/deg  RxUpperLimitDamping=10  RxUpperLimitDampingUnits=N*m/(deg/s)  RxUpperLimitTransitionRegionWidth=0.1  RxUpperLimitTransitionRegionWidthUnits=deg  RxPositionTargetSpecify=off  RxPositionTargetPriority=High  RxPositionTargetValue=0  RxPositionTargetValueUnits=deg  RxVelocityTargetSpecify=off  RxVelocityTargetPriority=High  RxVelocityTargetValue=0  RxVelocityTargetValueUnits=deg/s  RyEquilibriumPosition=0  RyEquilibriumPositionUnits=deg  RySpringStiffness=0  RySpringStiffnessUnits=N*m/deg  RyDampingCoefficient=0  RyDampingCoefficientUnits=N*m/(deg/s)  RyTorqueActuationMode=ComputedTorque  RyMotionActuationMode=InputMotion  RySensePosition=off  RySenseVelocity=off  RySenseAcceleration=off  RySenseTorqueForce=off  RySenseLowerLimitTorqueForce=off  RySenseUpperLimitTorqueForce=off  RyLowerLimitSpecify=off  RyLowerLimitBound=-90  RyLowerLimitBoundUnits=deg  RyLowerLimitStiffness=1e4  RyLowerLimitStiffnessUnits=N*m/deg  RyLowerLimitDamping=10  RyLowerLimitDampingUnits=N*m/(deg/s)  RyLowerLimitTransitionRegionWidth=0.1  RyLowerLimitTransitionRegionWidthUnits=deg  RyUpperLimitSpecify=off  RyUpperLimitBound=90  RyUpperLimitBoundUnits=deg  RyUpperLimitStiffness=1e4  RyUpperLimitStiffnessUnits=N*m/deg  RyUpperLimitDamping=10  RyUpperLimitDampingUnits=N*m/(deg/s)  RyUpperLimitTransitionRegionWidth=0.1  RyUpperLimitTransitionRegionWidthUnits=deg  RyPositionTargetSpecify=off  RyPositionTargetPriority=High  RyPositionTargetValue=0  RyPositionTargetValueUnits=deg  RyVelocityTargetSpecify=off  RyVelocityTargetPriority=High  RyVelocityTargetValue=0  RyVelocityTargetValueUnits=deg/s  RzEquilibriumPosition=0  RzEquilibriumPositionUnits=deg  RzSpringStiffness=0  RzSpringStiffnessUnits=N*m/deg  RzDampingCoefficient=0  RzDampingCoefficientUnits=N*m/(deg/s)  RzTorqueActuationMode=ComputedTorque  RzMotionActuationMode=InputMotion  RzSensePosition=off  RzSenseVelocity=off  RzSenseAcceleration=off  RzSenseTorqueForce=off  RzSenseLowerLimitTorqueForce=off  RzSenseUpperLimitTorqueForce=off  RzLowerLimitSpecify=off  RzLowerLimitBound=-90  RzLowerLimitBoundUnits=deg  RzLowerLimitStiffness=1e4  RzLowerLimitStiffnessUnits=N*m/deg  RzLowerLimitDamping=10  RzLowerLimitDampingUnits=N*m/(deg/s)  RzLowerLimitTransitionRegionWidth=0.1  RzLowerLimitTransitionRegionWidthUnits=deg  RzUpperLimitSpecify=off  RzUpperLimitBound=90  RzUpperLimitBoundUnits=deg  RzUpperLimitStiffness=1e4  RzUpperLimitStiffnessUnits=N*m/deg  RzUpperLimitDamping=10  RzUpperLimitDampingUnits=N*m/(deg/s)  RzUpperLimitTransitionRegionWidth=0.1  RzUpperLimitTransitionRegionWidthUnits=deg  RzPositionTargetSpecify=off  RzPositionTargetPriority=High  RzPositionTargetValue=0  RzPositionTargetValueUnits=deg  RzVelocityTargetSpecify=off  RzVelocityTargetPriority=High  RzVelocityTargetValue=0  RzVelocityTargetValueUnits=deg/s
  MATLAB Function2 : MATLAB Function  TreatAsAtomicUnit=on
  PS-Simulink Converter{,6..7,11..13} (6 alike) : nesl_utility/PS-Simulink Converter  PhysicalDomain=network_engine_domain  SubClassName=ps_output  LeftPortType=input  RightPortType=output  PseudoPeriodic=off  Frequencies=[]  VectorFormat=inherit  Unit=inherit  AffineConversion=off
  Simulink-PS Converter : nesl_utility/Simulink-PS Converter  PhysicalDomain=network_engine_domain  SubClassName=ps_input  LeftPortType=input  RightPortType=output  PseudoPeriodic=off  Frequencies=[]  NoiseDistribution=none  NoiseParameters=[]  Unit=m  AffineConversion=off  FilteringAndDerivatives=provide  SimscapeFilterOrder=1  InputFilterTimeConstant=0.001  UdotUserProvided=0
  Simulink-PS Converter10 : nesl_utility/Simulink-PS Converter  PhysicalDomain=network_engine_domain  SubClassName=ps_input  LeftPortType=input  RightPortType=output  PseudoPeriodic=off  Frequencies=[]  NoiseDistribution=none  NoiseParameters=[]  Unit=1  AffineConversion=off  FilteringAndDerivatives=provide  SimscapeFilterOrder=2  InputFilterTimeConstant=0.001  UdotUserProvided=2
  Simulink-PS Converter11 : nesl_utility/Simulink-PS Converter  PhysicalDomain=network_engine_domain  SubClassName=ps_input  LeftPortType=input  RightPortType=output  PseudoPeriodic=off  Frequencies=[]  NoiseDistribution=none  NoiseParameters=[]  Unit=1  AffineConversion=off  FilteringAndDerivatives=provide  SimscapeFilterOrder=2  InputFilterTimeConstant=0.001  UdotUserProvided=2
  Simulink-PS Converter9 : nesl_utility/Simulink-PS Converter  PhysicalDomain=network_engine_domain  SubClassName=ps_input  LeftPortType=input  RightPortType=output  PseudoPeriodic=off  Frequencies=[]  NoiseDistribution=none  NoiseParameters=[]  Unit=1  AffineConversion=on  FilteringAndDerivatives=provide  SimscapeFilterOrder=2  InputFilterTimeConstant=0.1  UdotUserProvided=2
  Transform Sensor : sm_lib/Frames and Transforms/Transform Sensor  MeasurementFrame=Base  RotationSequence=XYZ  SenseAngle=off  SenseAxis=off  SenseQ=off  SenseR=off  SenseRotationSequence=off  SenseOmegaX=off  SenseOmegaY=off  SenseOmegaZ=off  SenseQDot=off  SenseRDot=off  SenseRotationSequenceDot=off  SenseAlphaX=off  SenseAlphaY=off  SenseAlphaZ=off  SenseQDDot=off  SenseRDDot=off  SenseX=on  SenseY=on  SenseZ=on  SenseRad=off  SenseAzim=off  SenseDist=off  SenseInc=off  SenseXDot=off  SenseYDot=off  SenseZDot=off  SenseRadDot=off  SenseAzimDot=off  SenseDistDot=off  SenseIncDot=off  SenseXDDot=off  SenseYDDot=off  SenseZDDot=off  SenseRadDDot=off  SenseAzimDDot=off  SenseDistDDot=off  SenseIncDDot=off
  Transform Sensor1 : sm_lib/Frames and Transforms/Transform Sensor  MeasurementFrame=Base  RotationSequence=XYZ  SenseAngle=off  SenseAxis=off  SenseQ=off  SenseR=off  SenseRotationSequence=off  SenseOmegaX=off  SenseOmegaY=off  SenseOmegaZ=off  SenseQDot=off  SenseRDot=off  SenseRotationSequenceDot=off  SenseAlphaX=off  SenseAlphaY=off  SenseAlphaZ=off  SenseQDDot=off  SenseRDDot=off  SenseX=on  SenseY=on  SenseZ=on  SenseRad=off  SenseAzim=off  SenseDist=off  SenseInc=off  SenseXDot=off  SenseYDot=off  SenseZDot=off  SenseRadDot=off  SenseAzimDot=off  SenseDistDot=off  SenseIncDot=off  SenseXDDot=off  SenseYDDot=off  SenseZDDot=off  SenseRadDDot=off  SenseAzimDDot=off  SenseDistDDot=off  SenseIncDDot=off
  Transport Delay : TransportDelay  DelayTime=1e-6
  Transport Delay1 : TransportDelay  DelayTime=1e-6
  Transport Delay2 : TransportDelay  DelayTime=1e-6
  Variable Cylindrical Solid : sm_lib/Body Elements/Variable Mass/Variable Cylindrical Solid  LengthType=ProvidedByInput  Length=1  LengthUnits=m  RadiusType=Constant  Radius=muscle_radius  RadiusUnits=mm  MassType=CalculateFromGeometry  InitialMassType=Specified  InitialMass=1  InitialMassUnits=kg  Density=0.1  DensityUnits=kg/m^3  SenseRadius=off  SenseLength=off  SenseMass=off  SenseCenterOfMass=off  SenseInertiaMatrix=off  GraphicType=FromGeometry  MarkerShape=Sphere  MarkerSize=10  GraphicVisPropType=SimpleVisualProperties  GraphicDiffuseColor=muscle_color  GraphicSpecularColor=[0.5 0.5 0.5 1.0]  GraphicAmbientColor=[0.15 0.15 0.15 1.0]  GraphicEmissiveColor=[0.0 0.0 0.0 1.0]  GraphicShininess=75  GraphicOpacity=1.0
  MuscleEnd1 : PMIOPort  Side=Right
  MuscleEnd2 : PMIOPort  Port=2  Side=Right
  R : PMIOPort  Port=3  Side=Right
  wires:
  Constant1/1 -> Simulink-PS Converter9/3, Simulink-PS Converter10/3, Simulink-PS Converter11/3
  Constant/1 -> Simulink-PS Converter9/2, Simulink-PS Converter10/2, Simulink-PS Converter11/2
  MATLAB Function2/1(length) -> Simulink-PS Converter/1
  PS-Simulink Converter6/1 -> MATLAB Function2/2(y1)
  PS-Simulink Converter12/1 -> MATLAB Function2/5(y2)
  Transport Delay2/1 -> Simulink-PS Converter11/1
  MATLAB Function2/2(Rx) -> Transport Delay1/1
  MATLAB Function2/3(Ry) -> Transport Delay/1
  PS-Simulink Converter/1 -> MATLAB Function2/1(x1)
  PS-Simulink Converter13/1 -> MATLAB Function2/6(z2)
  Transport Delay1/1 -> Simulink-PS Converter9/1
  PS-Simulink Converter11/1 -> MATLAB Function2/4(x2)
  MATLAB Function2/4(Rz) -> Transport Delay2/1
  Transport Delay/1 -> Simulink-PS Converter10/1
  PS-Simulink Converter7/1 -> MATLAB Function2/3(z1)
  connections:
  MuscleEnd2/RConn1 -- Transform Sensor1/RConn1
  Simulink-PS Converter/RConn1 -- Variable Cylindrical Solid/LConn1
  Transform Sensor1/RConn3 -- PS-Simulink Converter12/LConn1
  Transform Sensor1/LConn1 -- R/RConn1 -- Transform Sensor/LConn1
  Transform Sensor1/RConn4 -- PS-Simulink Converter13/LConn1
  Transform Sensor/RConn2 -- PS-Simulink Converter/LConn1
  Transform Sensor/RConn3 -- PS-Simulink Converter6/LConn1
  Transform Sensor/RConn1 -- MuscleEnd1/RConn1 -- Gimbal Joint/LConn1
  Transform Sensor1/RConn2 -- PS-Simulink Converter11/LConn1
  Gimbal Joint/RConn1 -- Variable Cylindrical Solid/RConn1
  Simulink-PS Converter11/RConn1 -- Gimbal Joint/LConn4
  Simulink-PS Converter10/RConn1 -- Gimbal Joint/LConn3
  Transform Sensor/RConn4 -- PS-Simulink Converter7/LConn1
  Simulink-PS Converter9/RConn1 -- Gimbal Joint/LConn2
